simulink model "CompleteDronePathSimulation2"  (R2022b)
settings: Solver=VariableStepAuto  StartTime=0.0  StopTime=10.0  RelTol=1e-3
settings Model: Creator=zs  LastModifiedBy=zs

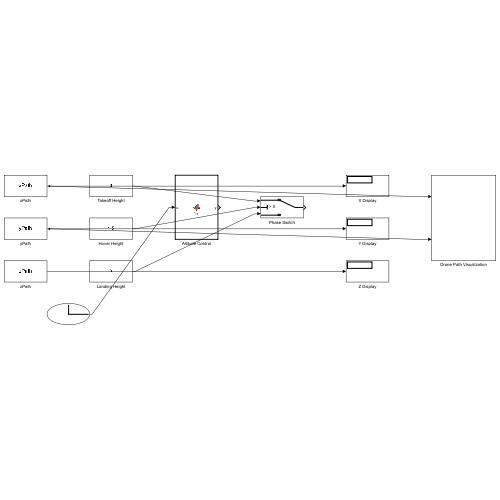
[thumbnail: Simulink's stored preview of the top-level diagram]
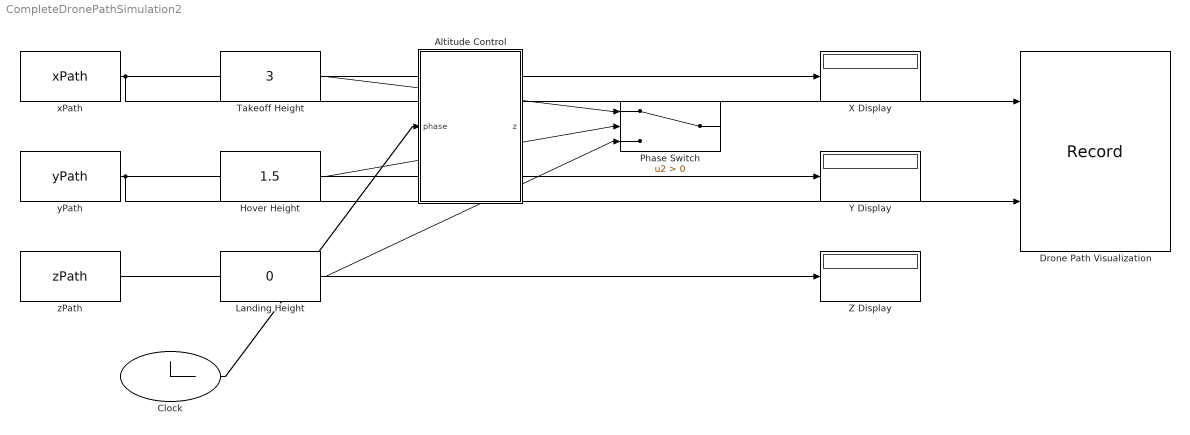
== system CompleteDronePathSimulation2 ==
  Altitude Control : MATLAB Function  TreatAsAtomicUnit=on
  Clock : Clock
  Drone Path Visualization : Record  FileSettingsInternal="{\"entries\":[{\"content\":{\"excelSettings\":{\"content\":{},\"type\":\"Streamout.ExcelSettings\"}},\"type\":\"Streamout.FileSettingStorage\",\"uuid\":\"f0656e0d-14b3-4b35-a4d4-bfa3119b52c7\"}],\"packageUris\":[\"http://schema.mathworks.com/mf0/streamout_blocks/R2020a\"],\"version\":\"1.0\"}"  Layout=[1 1]  SignalsInternal="{\"entries\":[{\"content\":{\"signals\":[{\"content\":{\"blockPath\":[\"CompleteDronePathSimulation2/Drone Path Visualization\"],\"channel\":[],\"dimensions\":[1],\"domain\":\"CompleteDronePathSimulation2/Drone Path Visualization\",\"lineColor\":\"#a2142f\",\"plots\":[1],\"port\":1,\"sid\":[],\"signalID\":915,\"signalName\":\"XY Graph:1\"},\"type\":\"RecordBlkView.Signal\",\"uuid\":\"5e88ab2b-473f-48de-9c82-a0928789c8fe\"},{\"content\":{\"blockPath\":[\"CompleteDronePathSimulation2/Drone Path Visualization\"],\"channel\":[],\"dimensions\":[1],\"domain\":\"CompleteDronePathSimulation2/Drone Path Visualization\",\"lineColor\":\"#139fff\",\"plots\":[1],\"port\":2,\"sid\":[],\"signalID\":918,\"signalName\":\"XY Graph:2\"},\"type\":\"RecordBlkView.Signal\",\"uuid\":\"762bb7ac-2f74-4699-84e8-45141038c420\"}]},\"type\":\"RecordBlkView.InputSignals\",\"uuid\":\"b593c166-f5da-4a35-9326-b8c3075682d2\"}],\"packageUris\":[\"http://schema.mathworks.com/mf0/streamout_blocks/R2020a\"],\"version\":\"1.0\"}"  VisualizationBindings="{\"xyplotplugin\":{\"info\":[{\"series\":[{\"bindingParametersList\":[{\"parameter\":\"X-Axis\",\"signalID\":915,\"signalName\":\"XY Graph:1\"},{\"parameter\":\"Y-Axis\",\"signalID\":918,\"signalName\":\"XY Graph:2\"}],\"seriesID\":5391}],\"subplotID\":1}]}}"  CompatibilityTag=XY
  Hover Height : Constant  Value=1.5
  Landing Height : Constant  Value=0
  Phase Switch : Switch  Criteria=u2 > Threshold  SaturateOnIntegerOverflow=off  InputSameDT=off
  Takeoff Height : Constant  Value=3
  X Display : Display
  Y Display : Display
  Z Display : Display
  xPath : FromWorkspace  VariableName=xPath
  yPath : FromWorkspace  VariableName=yPath
  zPath : FromWorkspace  VariableName=zPath
  wires:
  xPath/1 -> X Display/1, Drone Path Visualization/1
  yPath/1 -> Y Display/1, Drone Path Visualization/2
  zPath/1 -> Z Display/1
  Clock/1 -> Altitude Control/1(phase)
  Takeoff Height/1 -> Phase Switch/1
  Hover Height/1 -> Phase Switch/2
  Landing Height/1 -> Phase Switch/3

== matlab function CompleteDronePathSimulation2/Altitude Control ==
  data: phase input; z output
function z = fcn(phase)
    if phase == 1
        z = 3;       % Takeoff height
    elseif phase == 2
        z = 1.5;     % Hover height
    else
        z = 0;       % Landing height
    end
end
